simulink model "custom_bouncing_ball"  (R2021b)
settings: Solver=FixedStepAuto  StartTime=0.0  StopTime=10.0  RelTol=1e-3
PreLoadFcn:
  | init
values from neighbouring files (symbols this model uses):
  g = 9.81    [sldemo_bounceExample.m]
undefined symbols (not defined in the file or in its folder): r, v
settings Model: Creator=lordx  LastModifiedBy=lordx
settings OptimizationCC: OptimizeBlockIOStorage=off  OptimizeDataStoreBuffers=off  BusAssignmentInplaceUpdate=off
settings DebuggingCC: SFUnexpectedBacktrackingDiag=warning  SFNoUnconditionalDefaultTransitionDiag=warning
settings HardwareCC: TargetBitPerPointer=64  TargetBitPerSizeT=64  TargetBitPerPtrDiffT=64  TargetLongLongMode=on  TargetIntDivRoundTo=Zero  TargetEndianess=LittleEndian  TargetWordSize=64  TargetHWDeviceType=MATLAB Host  ProdEqTarget=off
settings RTWCC: Description=FMU based on GRT (Functional Mock-up Unit)  SystemTargetFile=grtfmi.tlc  GenerateMakefile=off  TemplateMakefile=none  GenerateReport=on  RetainRTWFile=on  Toolchain=AUTOSAR Adaptive | CMake  BuildConfiguration=Debug  LaunchReport=on
settings CodeAppCC: ForceParamTrailComments=on  StateflowObjectComments=on  MATLABSourceComments=on  EnableCustomComments=on
settings STFCustomTargetCC: TargetLangStandard=C99 (ISO)  CombineOutputUpdateFcns=on  GRTInterface=off  SystemTargetFile=grtfmi.tlc
settings GRTTargetCC: ParMdlRefBuildCompliant=off  CompOptLevelCompliant=off  ConcurrentExecutionCompliant=off  MatFileLogging=off  CPPClassGenCompliant=off  UseToolchainInfoCompliant=off  RTWCAPISignals=on  RTWCAPIParams=on  RTWCAPIStates=on  RTWCAPIRootIO=on

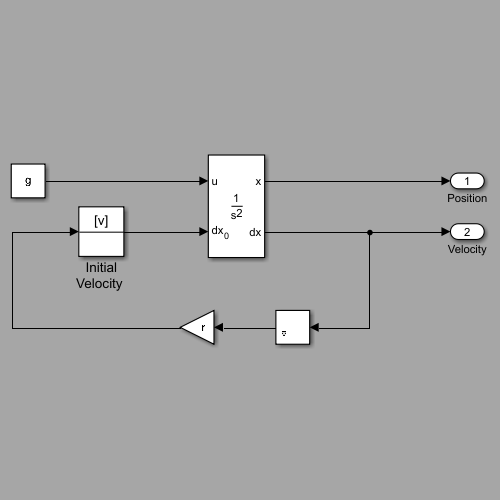
[thumbnail: Simulink's stored preview of the top-level diagram]
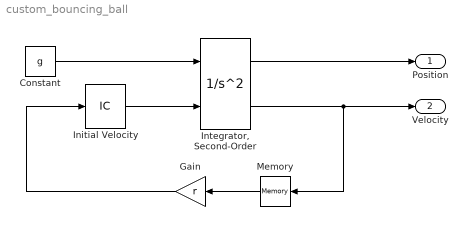
== system custom_bouncing_ball ==
  Constant : Constant  Value=g
  Gain : Gain  Gain=r
  "Initial Velocity " : InitialCondition  Value=v
  "Integrator, Second-Order" : SecondOrderIntegrator  ICSourceDXDT=external
  Memory : Memory
  Position : Outport
  Velocity : Outport  Port=2
  wires:
  "Initial Velocity "/1 -> "Integrator, Second-Order"/2
  Constant/1 -> "Integrator, Second-Order"/1
  "Integrator, Second-Order"/2 -> Memory/1, Velocity/1
  "Integrator, Second-Order"/1 -> Position/1
  Memory/1 -> Gain/1
  Gain/1 -> "Initial Velocity "/1
